simulink model "ee464_hw_project1"  (R2021b)
settings: Solver=VariableStepAuto  StartTime=0.0  StopTime=1  RelTol=1e-3
libraries: spsSeriesRLCBranchLib x3, spsRMSLib x3, spsCurrentMeasurementLib x2, spsDiodeLib x2, spsIdealSwitchLib x2, spsVoltageMeasurementLib x2, spsLinearTransformerLib x1, spsPWMGeneratorDCDCLib x1, spsParallelRLCBranchLib x1, spsDCVoltageSourceLib x1, spspowerguiLib x1
settings Model: Creator=ASUS  LastModifiedBy=Emre Çakmakyurdu
settings SolverCC: ZeroCrossAlgorithm=Adaptive
settings OptimizationCC: DefaultParameterBehavior=Inlined  EnhancedBackFolding=on  PassReuseOutputArgsAs=Individual arguments  ZeroExternalMemoryAtStartup=off  ZeroInternalMemoryAtStartup=off  OptimizeBlockOrder=speed  DifferentSizesBufferReuse=on  OptimizationCustomize=off  EfficientTunableParamExpr=on
settings DebuggingCC: IgnoredZcDiagnostic=none  ParameterTunabilityLossMsg=error
settings SFSimCC: MATLABDynamicMemAlloc=off
settings RTWCC: Description=Embedded Coder  SystemTargetFile=ert.tlc  TemplateMakefile=ert_default_tmf
settings CodeAppCC: ForceParamTrailComments=on  IgnoreCustomStorageClasses=off  OperatorAnnotations=on  SimulinkDataObjDesc=on  SFDataObjDesc=on  InsertBlockDesc=on
settings ERTTargetCC: TargetLangStandard=C99 (ISO)  GenerateSampleERTMain=on  InlinedParameterPlacement=NonHierarchical  ERTCustomFileTemplate=example_file_process.tlc

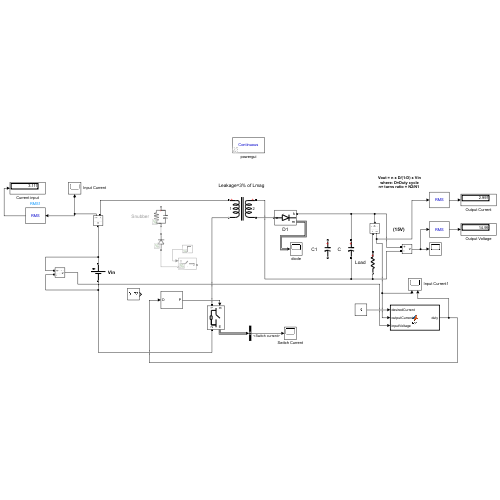
[thumbnail: Simulink's stored preview of the top-level diagram]
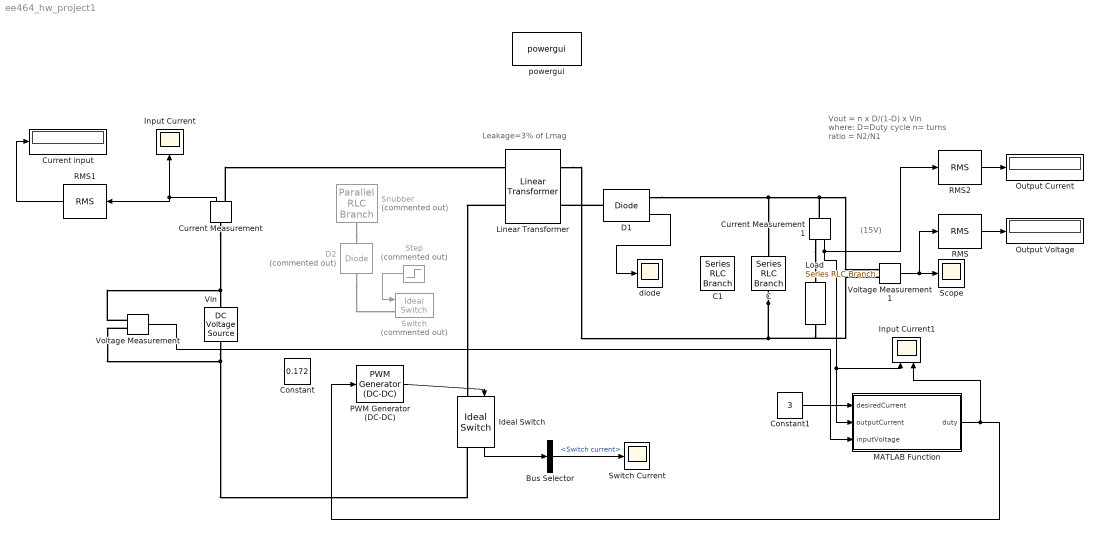
== system ee464_hw_project1 ==
  note: Leakage=3% of Lmag
  note: Vout = n x D/(1-D) x Vin
      | where: D=Duty cycle
      | n= turns ratio = N2/N1
  note: (15V)
  Bus Selector : BusSelector  OutputSignals=Switch current
  C : spsSeriesRLCBranchLib/Series RLC Branch  LConnTagsString=__new0  RConnTagsString=__new0  BranchType=C  Resistance=1e-4  Inductance=200e-6  SetiL0=off  InitialCurrent=0  Capacitance=50e-6  Setx0=off  InitialVoltage=0  Measurements=None
  C1 : spsSeriesRLCBranchLib/Series RLC Branch  LConnTagsString=__new0  RConnTagsString=__new0  BranchType=C  Resistance=1e-4  Inductance=200e-6  SetiL0=off  InitialCurrent=0  Capacitance=0.5e-6  Setx0=off  InitialVoltage=0  Measurements=None
  Constant : Constant  Value=0.172
  Constant1 : Constant  Value=3
  Current Measurement : spsCurrentMeasurementLib/Current Measurement  PhasorSimulation=off  OutputType=Complex  PSBequivalent=0
  Current Measurement1 : spsCurrentMeasurementLib/Current Measurement  PhasorSimulation=off  OutputType=Complex  PSBequivalent=0
  Current input : Display
  D1 : spsDiodeLib/Diode  Ron=1e-3  Lon=0  Vf=0  IC=0  UseSnubber=off  Rs=inf  Cs=0  Measurements=on
  D2 : spsDiodeLib/Diode  Commented=on  Ron=1e-3  Lon=0  Vf=0  IC=0  UseSnubber=off  Rs=inf  Cs=0  Measurements=off
  Ideal Switch : spsIdealSwitchLib/Ideal Switch  Ron=0.001  Lon=0  IC=0  Rs=1e5  Cs=inf  Measurements=on
  Input Current : Scope
  Input Current1 : Scope  NumInputPorts=2
  Linear Transformer : spsLinearTransformerLib/Linear Transformer  UNITS=SI  NominalPower=[ 45 100e3 ]  winding1=[48 0 0]  winding2=[30 0 0]  ThreeWindings=off  winding3=[3.15e+05 3.969e+07 6316.9]  RmLm=[1e4 16e-6]  Measurements=Magnetization current  DataType=on
  Load : spsSeriesRLCBranchLib/Series RLC Branch  LConnTagsString=__new0  RConnTagsString=__new0  BranchType=R  Resistance=5  Inductance=200e-6  SetiL0=off  InitialCurrent=0  Capacitance=400e-6  Setx0=off  InitialVoltage=0  Measurements=Branch current
  MATLAB Function : MATLAB Function  TreatAsAtomicUnit=on
  Output Current : Display
  Output Voltage : Display
  PWM Generator (DC-DC) : spsPWMGeneratorDCDCLib/PWM Generator (DC-DC)  Fsw=100e3  Ts=0
  RMS : spsRMSLib/RMS  TrueRMS=on  Freq=60  RMSInit=0  Ts=0
  RMS1 : spsRMSLib/RMS  TrueRMS=on  Freq=60  RMSInit=0  Ts=0
  RMS2 : spsRMSLib/RMS  TrueRMS=on  Freq=60  RMSInit=0  Ts=0
  Scope : Scope
  Snubber : spsParallelRLCBranchLib/Parallel RLC Branch  Commented=on  LConnTagsString=a  RConnTagsString=__new0  BranchType=RC  Resistance=10e3  Inductance=1e-3  SetiL0=off  InitialCurrent=0  Capacitance=47e-9  Setx0=off  InitialVoltage=0  Measurements=None
  Step : Step  Commented=on  Time=0.00385  SampleTime=0
  Switch : spsIdealSwitchLib/Ideal Switch  Commented=on  Ron=0.001  Lon=0  IC=0  Rs=inf  Cs=0  Measurements=off
  Switch Current : Scope
  Vin : spsDCVoltageSourceLib/DC Voltage Source  Amplitude=24  Measurements=None
  Voltage Measurement : spsVoltageMeasurementLib/Voltage Measurement  PhasorSimulation=off  OutputType=Complex  PSBequivalent=0
  Voltage Measurement1 : spsVoltageMeasurementLib/Voltage Measurement  PhasorSimulation=off  OutputType=Complex  PSBequivalent=0
  diode : Scope
  powergui : spspowerguiLib/powergui  Priority=1  SimulationMode=Continuous  SampleTime=1e-5  frequency=60  Iterations=50  frequencyindice=0  Pbase=100e6  ErrMax=1e-4  UnitsV=kV  UnitsW=MW  buscounter=0  FunctionMessages=off  echomessages=off  EnableUseOfTLC=off  CurrentSourceSwitches=off  DisableSnubberDevices=off  DisableRonSwitches=off  DisableVfSwitches=off  DisplayEquations=off  AutomaticDiscreteSolvers=off  SolverType=Tustin/Backward Euler (TBE)  Interpol=off  ExternalGateDelay=off  methode=off  Ts=100  x0status=blocks  SPID=on  SwTol=0  HookPort=off  NonlinearTolerance=1e-4  nMaxIteration=100  ContinueOnMaxIteration=off  RestoreLinks=warning  ResistiveCurrentMeasurement=off  Frange=[0:2:500]  Ylog=off  Xlog=on  ShowGrid=off  save=off  variable=ZData  structure=0  ZoomFFT=off  StartTime=0.0  cycles=1  DisplayStyle=1  fundamental=60  FreqAxis=off  MaxFrequency=1000  frequencyindicesteady=1  RmsSteady=1  display=off
  wires:
  D1/1 -> diode/1
  Step/1 -> Switch/1
  Voltage Measurement1/1 -> RMS/1, Scope/1
  PWM Generator (DC-DC)/1 -> Ideal Switch/1
  Ideal Switch/1 -> Bus Selector/1
  Bus Selector/1 -> Switch Current/1  "<Switch current>"
  Current Measurement/1 -> Input Current/1, RMS1/1
  Constant1/1 -> MATLAB Function/1(desiredCurrent)
  Current Measurement1/1 -> Input Current1/1, MATLAB Function/2(outputCurrent), RMS2/1
  MATLAB Function/1(duty) -> PWM Generator (DC-DC)/1, Input Current1/2
  Voltage Measurement/1 -> MATLAB Function/3(inputVoltage)
  RMS/1 -> Output Voltage/1
  RMS1/1 -> Current input/1
  RMS2/1 -> Output Current/1
  connections:
  Current Measurement/RConn1 -- Linear Transformer/LConn1
  C/RConn1 -- Linear Transformer/RConn1 -- Load/RConn1 -- Voltage Measurement1/LConn2
  Linear Transformer/LConn2 -- Ideal Switch/LConn1
  D1/RConn1 -- Current Measurement1/LConn1 -- Voltage Measurement1/LConn1 -- C/LConn1
  D2/LConn1 -- Switch/LConn1
  Snubber/RConn1 -- D2/RConn1
  Vin/LConn1 -- Ideal Switch/RConn1 -- Voltage Measurement/LConn2
  D1/LConn1 -- Linear Transformer/RConn2
  Current Measurement/LConn1 -- Voltage Measurement/LConn1 -- Vin/RConn1
  Current Measurement1/RConn1 -- Load/LConn1

== matlab function ee464_hw_project1/MATLAB Function ==
  settings: updateMethod=DISCRETE
  data: desiredCurrent input; duty output; outputCurrent input; inputVoltage input
function duty = fcn(desiredCurrent , outputCurrent, inputVoltage)
    
    persistent difference
    if isempty(difference)
        difference = 0;
    end
    duty = 9.375/(9.375 + inputVoltage) + difference/5.6;
    difference = desiredCurrent - outputCurrent;
    if(inputVoltage <= 48 && inputVoltage >40)
        duty = 9.375/(9.375 + inputVoltage) + difference/4.7;
    end
    if(inputVoltage <= 36 && inputVoltage > 24)
        duty = 9.375/(9.375 + inputVoltage) + difference/6;
    end
    
end
